simulink model "IID_nms_2Dmodel_for"  (R2016b)
settings: Solver=ode15s  StartTime=0.0  StopTime=t_end  FixedStep=1e-3  MaxStep=ts_max  RelTol=1e-3  AbsTol=1e-4  EnableMultiTasking=on
InitFcn:
  | IID_runScripts;
values from neighbouring files (symbols this model uses):
  D12_F = 0.16    [IID_nms_MechInit.m]    (also in nms_MechInit.m)
  D12_S = L_S    (= 0.5)    [IID_nms_MechInit.m]    (also in nms_MechInit.m = 0.46)
  D12_T = L_T    (= 0.5)    [IID_nms_MechInit.m]    (also in nms_MechInit.m = 0.46)
  D13_F = 0.20    (= 0.2)    [IID_nms_MechInit.m]    (also in nms_MechInit.m)
  D1G_F = 0.14    [IID_nms_MechInit.m]    (also in nms_MechInit.m)
  D1G_HAT = 0.35    [IID_nms_MechInit.m]    (also in nms_MechInit.m)
  D1G_S = 0.3    [IID_nms_MechInit.m]    (also in nms_MechInit.m = 0.28)
  D1G_T = 0.3    [IID_nms_MechInit.m]    (also in nms_MechInit.m = 0.28)
  DeltaThRef = 5e-3    (= 0.005)    [IID_nms_MechInit.m]    (also in nms_MechInit.m)
  Dist_On = 1    [IID_setDistPar.m]    (also in setDistPar.m)
  Dist_PDur = 0.15    [IID_setDistPar.m]    (also in setDistPar.m)
  Dist_StartTime = 15    [IID_setDistPar.m]    (also in setDistPar.m)
  Dist_xyzHAT_sag_PH = 0    [IID_setDistPar.m]    (also in setDistPar.m)
  In_F = 0.005    [IID_nms_MechInit.m]    (also in nms_MechInit.m)
  In_HAT = 3    [IID_nms_MechInit.m]    (also in nms_MechInit.m = 2.5)
  In_S = 0.05    [IID_nms_MechInit.m]    (also in nms_MechInit.m)
  In_T = 0.15    [IID_nms_MechInit.m]    (also in nms_MechInit.m)
  k_gx = (2*(m_F+m_S+m_T)+m_HAT)*g/0.1    (= 7848)    [IID_nms_MechInit.m]
  k_gy = (2*(m_F+m_S+m_T)+m_HAT)*g/0.01    (= 78480)    [IID_nms_MechInit.m]
  k_pressure = m_HAT * 9.81 / DeltaThRef    (= 104967)    [IID_nms_MechInit.m]    (also in nms_MechInit.m)
  m_F = 1.25    [IID_nms_MechInit.m]    (also in nms_MechInit.m)
  m_HAT = 53.5    [IID_nms_MechInit.m]    (also in nms_MechInit.m)
  m_S = 3.5    [IID_nms_MechInit.m]    (also in nms_MechInit.m)
  m_T = 8.5    [IID_nms_MechInit.m]    (also in nms_MechInit.m)
  m_Total = m_F*2+m_S*2+m_T*2+m_HAT    (= 80)    [IID_nms_MechInit.m]    (also in nms_MechInit.m)
  MidDelay = 0.010    (= 0.01)    [IID_setCtrlPar.m]    (also in nms_MechInit.m = 0.005)
  mu_slide = 0.8    [IID_nms_MechInit.m]    (also in nms_MechInit.m)
  mu_stick = 0.9    [IID_nms_MechInit.m]    (also in nms_MechInit.m)
  N = 1.5    [IID_nms_MechInit.m]    (also in cmaes_parfor.m = size(x,1); nms_MechInit.m)
  s = x(1:N-1,:).^2 + x(2:N,:).^2    [cmaes_parfor.m]
  ThPos = 4/5    (= 0.8)    [IID_nms_MechInit.m]    (also in nms_MechInit.m)
  v_gx_max = 0.03    [IID_nms_MechInit.m]
  v_gy_max = 0.03    [IID_nms_MechInit.m]
  v_max_pressure = 0.5    [IID_nms_MechInit.m]    (also in nms_MechInit.m)
  vLimit = 0.01    [IID_nms_MechInit.m]    (also in nms_MechInit.m)
undefined symbols (not defined in the file or in its folder): sgn
libraries: mblibv1 x71, cpg_lib x23, simulink x21, simulink_extras x6
(part 1 of 3)
settings Model: SimulationMode=accelerator  Creator=hgeyer  LastModifiedBy=brugtjh
settings SolverCC: ZeroCrossControl=DisableAll
settings DataIOCC: SaveFormat=Array  SignalLoggingSaveFormat=ModelDataLogs  SignalLogging=off
settings OptimizationCC: BooleanDataType=off  ExpressionDepthLimit=2147483647  InitFltsAndDblsToZero=on  EfficientMapNaN2IntZero=off  LifeSpan=inf
settings DebuggingCC: SaveWithParameterizedLinksMsg=none  UnderspecifiedInitializationDetection=Classic  MergeDetectMultiDrivingBlocksExec=none  SignalResolutionControl=TryResolveAllWithWarning  SolverPrmCheckMsg=warning  MultiTaskDSMMsg=warning  MultiTaskCondExecSysMsg=none  FcnCallInpInsideContextMsg=warning  AllowSymbolicDim=off  StateNameClashWarn=warning  SFUnexpectedBacktrackingDiag=warning  SFNoUnconditionalDefaultTransitionDiag=warning  SFExecutionAtInitializationDiag=none
settings HardwareCC: ProdBitPerPointer=32  ProdBitPerSizeT=32  ProdBitPerPtrDiffT=32  ProdLargestAtomicFloat=None  ProdIntDivRoundTo=Undefined  ProdEndianess=Unspecified  ProdWordSize=32  ProdHWDeviceType=32-bit Generic  TargetBitPerPointer=64  TargetBitPerSizeT=64  TargetBitPerPtrDiffT=64  TargetLongLongMode=on  TargetIntDivRoundTo=Zero  TargetEndianess=LittleEndian  TargetWordSize=64  TargetHWDeviceType=MATLAB Host  ProdEqTarget=off
settings ModelReferenceCC: PropagateSignalLabelsOutOfModel=off
settings CodeAppCC: MaxIdLength=128
settings GRTTargetCC: TargetLangStandard=C89/C90 (ANSI)  CombineOutputUpdateFcns=off  GRTInterface=on
settings ConfigComp: CovMetricSettings=dw  CovHtmlReporting=on  CovSaveCumulativeToWorkspaceVar=on  CovSaveSingleToWorkspaceVar=on  CovExternalEMLEnable=off
settings ConfigurationSet: Description=SimMechanics 2G
settings ExplorerConfigSet: SimMechanicsOpenEditorOnUpdate=off

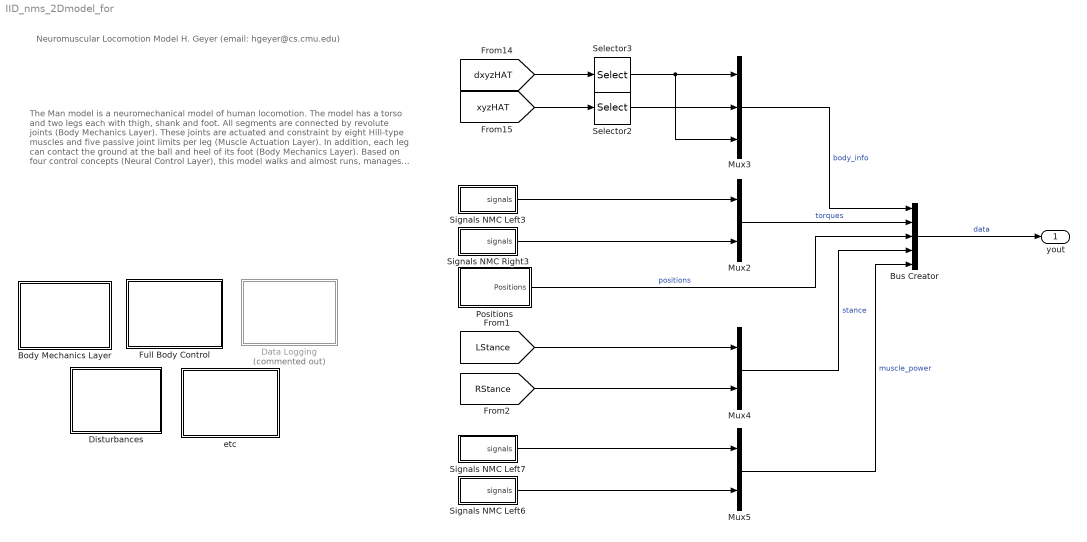
== system IID_nms_2Dmodel_for ==
  note: The Man model is a neuromechanical model of human locomotion.
      | The model has a torso and two legs each with thigh, shank and
      | foot. All segments are connected by revolute joints (Body Mechanics
      | Layer). These joints are actuated and constraint by eight Hill-type
      | muscles and five passive joint limits per leg (Muscle Actuation Layer).
      | In addition, each leg can contact the ground at the ball and heel of
      | its foot (Body Mechanics Layer).
      |
      | Based on four control concepts (Neural Control Layer), this
      | model walks and almost runs, manages slopes and random ground
      | levels, and adapts to different surfaces.
  note: Neuromuscular Locomotion Model
      | H. Geyer
      | (email: hgeyer@cs.cmu.edu)
  Body Mechanics Layer : Subsystem
  Bus Creator : BusCreator  Inputs=5
  Data Logging : Subsystem  Commented=on
  Disturbances : Subsystem
  Full Body Control : Subsystem
  Mux2 : Mux  Inputs=2
  Mux3 : Mux  Inputs=3
  Mux4 : Mux  Inputs=2
  Mux5 : Mux  Inputs=2
  Positions : Subsystem
  Selector2 : Selector  InputPortWidth=3  IndexOptions=Index vector (dialog)  Indices=[1]  OutputSizes=1
  Selector3 : Selector  InputPortWidth=3  IndexOptions=Index vector (dialog)  Indices=[1]  OutputSizes=1
  Signals NMC Left3 : Subsystem
  Signals NMC Left6 : Subsystem
  Signals NMC Left7 : Subsystem
  Signals NMC Right3 : Subsystem
  etc : Subsystem
  yout : Outport
  wires:
  Bus Creator/1 -> yout/1  "data"
  Selector3/1 -> Mux3/3, Mux3/1
  [dxyzHAT] -> Selector3/1
  [xyzHAT] -> Selector2/1
  Selector2/1 -> Mux3/2
  Mux3/1 -> Bus Creator/1  "body_info"
  Signals NMC Left3/1(signals) -> Mux2/1
  Signals NMC Right3/1(signals) -> Mux2/2
  Mux2/1 -> Bus Creator/2  "torques"
  Positions/1(Positions) -> Bus Creator/3  "positions"
  [LStance] -> Mux4/1
  [RStance] -> Mux4/2
  Mux4/1 -> Bus Creator/4  "stance"
  Signals NMC Left6/1(signals) -> Mux5/2
  Signals NMC Left7/1(signals) -> Mux5/1
  Mux5/1 -> Bus Creator/5  "muscle_power"

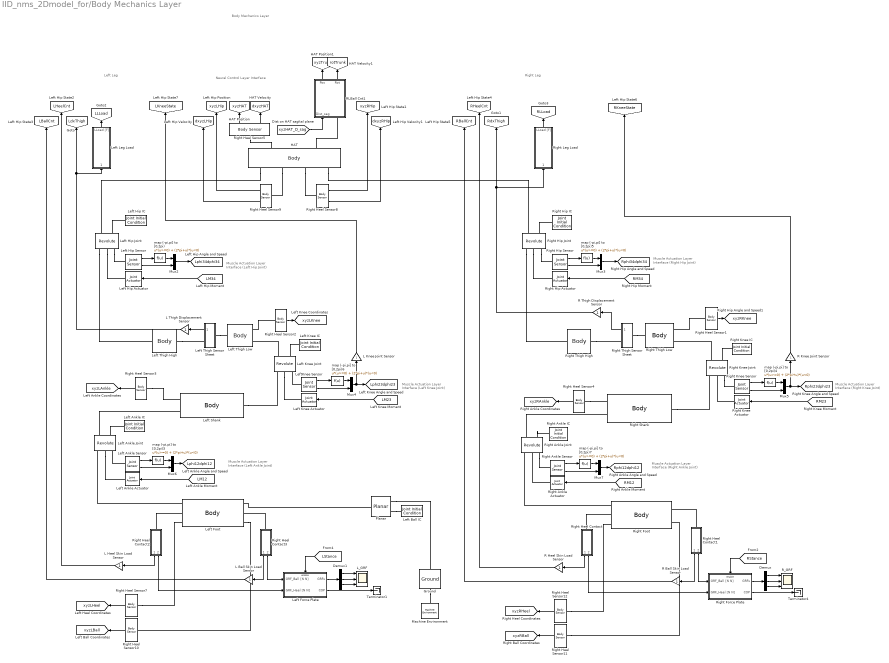
== system IID_nms_2Dmodel_for/Body Mechanics Layer ==
  note: Body Mechanics Layer
  note: Left Leg
  note: Right Leg
  note: Muscle Actuation
      | Layer Interface
      | (Left Hip Joint)
  note: Muscle Actuation
      | Layer Interface
      | (Right Hip Joint)
  note: Muscle Actuation
      | Layer Interface
      | (Right Knee Joint)
  note: Muscle Actuation
      | Layer Interface
      | (Left Knee Joint)
  note: Muscle Actuation
      | Layer Interface
      | (Left Ankle Joint)
  note: Muscle Actuation
      | Layer Interface
      | (Right Ankle Joint)
  note: Neural Control Layer Interface
  Demux : Demux  Outputs=3
  Demux1 : Demux  Outputs=3
  Ground : mblibv1/Bodies/Ground  UpdateFromCAD=off  LeftPortType=env  RightPortType=workingframe  PhysicalDomain=Mechanical  DialogClass=GroundBlock  CoordPosition=[0 0 0]  CoordPositionUnits=m  StateVectorMgrId=-1  MachineId=[0 0]  ShowEnvPort=on  ParameterChecksum=[3274320975, 1670571099, 3302951954, 713231611]  TopologyChecksum=[2253370739, 2650906436, 1237763067, 2817762160]
  HAT : mblibv1/Bodies/Body  LConnTagsString=CG|CS6  RConnTagsString=CS1|CS2|CS3|CS4  UpdateFromCAD=off  DialogClass=MechanicalBodyBlock  Mass=m_HAT  MassUnits=kg  InertiaUnits=kg*m^2  Inertia=In_HAT*[0 0 0; 0 0 0; 0 0 1]  Shape=Cylinder  ShapeDims=[1 1]  ShapeUnits=m  ShapeUse=false  Density=1  DensityUnits=kg/m^3  DensityUse=false  GraphicsMode=MACHINE_DEFAULT  BodyColorSelMode=MACHINE_DEFAULT  BodyColor=[1 0 0]  AttachedToCS=CG  CG=Left$CG$[D1G_HAT 0 0]$CS1$CS1$m$[0 0 0]$Euler X-Y-Z$deg$WORLD$true$none  WorkingFrames=Right$CS1$[0 0 0]$ADJOINING$ADJOINING$m$[0 0 0]$Euler X-Y-Z$deg$WORLD$true$none#Right$CS2$[0 0 0]$CS1$CS1$m$[0 0 0]$Euler X-Y-Z$deg$WORLD$true$none#Right$CS3$[0 0 0]$CS1$CS1$m$[0 0 0]$Euler X-Y-Z$deg$WORLD$true$none#Right$CS4$[0 0 0]$CS1$CS1$m$[0 0 0]$Euler X-Y-Z$deg$WORLD$true$none#Left$CS6$[0 0 0]$CS1$CS1$m$[0 0 0]$Euler X-Y-Z$deg$WORLD$true$none#Left$CS5$[2*D1G_HAT 0 0]$CS1$CS1$m$[0 0 0]$Euler X-Y-Z$deg$WORLD$false$none  CGPos=[D1G_HAT 0 0]  CGRot=[0 0 0]  CS0Pos=[]  CS0Rot=[]  CS1Pos=[0 0 0]  CS1Rot=[0 0 0]  CS2Pos=[0 0 0]  CS2Rot=[0 0 0]  CS3Pos=[0 0 0]  CS3Rot=[0 0 0]  CS4Pos=[0 0 0]  CS4Rot=[0 0 0]  CS5Pos=[2*D1G_HAT 0 0]  CS5Rot=[0 0 0]  CS6Pos=[0 0 0]  CS6Rot=[0 0 0]  CS7Pos=[]  CS7Rot=[]  CS8Pos=[]  CS8Rot=[]  CS9Pos=[]  CS9Rot=[]  CS10Pos=[]  CS10Rot=[]  CS11Pos=[]  CS11Rot=[]  CS12Pos=[]  CS12Rot=[]  CS13Pos=[]  CS13Rot=[]  CS14Pos=[]  CS14Rot=[]  CS15Pos=[]  CS15Rot=[]  CS16Pos=[]  CS16Rot=[]  CS17Pos=[]  CS17Rot=[]  CS18Pos=[]  CS18Rot=[]  CS19Pos=[]  CS19Rot=[]  CS20Pos=[]  CS20Rot=[]
  L Ball Skin Load Sensor : Gain
  L Heel Skin Load Sensor : Gain
  L Knee Joint Sensor : Gain
  L Thigh Displacement  Sensor : Gain
  L_GRF : Scope  NumInputPorts=3
  Left Ankle Joint : mblibv1/Joints/Revolute  LConnTagsString=__newl0|SA1|SA2  RConnTagsString=__newr0|SA1  UpdateFromCAD=off  NumSAPorts=3  CutJoint=off  MarkAsCut=off  Primitives=revolute  PrimitiveProps=R1$WORLD$[0 0 1]$revolute  DialogClass=JointBlock  R1Axis=[0 0 1]
  Left Hip Joint : mblibv1/Joints/Revolute  LConnTagsString=__newl0|SA1|SA2  RConnTagsString=__newr0|SA1  UpdateFromCAD=off  NumSAPorts=3  CutJoint=off  MarkAsCut=off  Primitives=revolute  PrimitiveProps=R1$WORLD$[0 0 1]$revolute  DialogClass=JointBlock  R1Axis=[0 0 1]
  Left Knee Joint : mblibv1/Joints/Revolute  LConnTagsString=__newl0|SA1|SA2  RConnTagsString=__newr0|SA1  UpdateFromCAD=off  NumSAPorts=3  CutJoint=off  MarkAsCut=off  Primitives=revolute  PrimitiveProps=R1$WORLD$[0 0 -1]$revolute  DialogClass=JointBlock  R1Axis=[0 0 -1]
  Left Ankle Actuator : mblibv1/Sensors &  Actuators/Joint Actuator  UpdateFromCAD=off  PhysicalDomain=Mechanical  PortType=blob  ActuationStyle=Force  AngleUnits=deg  ArcVelocityUnits=deg/s  ArcAccelerationUnits=deg/s^2  CoordPositionUnits=m  VelocityUnits=m/s  AccelerationUnits=m/s^2  ForceUnits=N  TorqueUnits=N-m  ActiveIO=on  Width=1  DialogClass=MechanicalActuatorBlock  Primitive=R1  ReferenceFrame=Absolute (INERTIAL)
  Left Ankle Sensor : mblibv1/Sensors &  Actuators/Joint Sensor  UpdateFromCAD=off  PhysicalDomain=Mechanical  PortType=blob  Muxed=off  Pose=off  Angle=on  AngleUnits=rad  ArcVelocity=on  ArcVelocityUnits=rad/s  ArcAcceleration=off  ArcAccelerationUnits=deg/s^2  CoordPosition=on  CoordPositionUnits=m  Velocity=off  VelocityUnits=m/s  Acceleration=off  AccelerationUnits=m/s^2  Quaternion=on  QuaternionDT=off  QuaternionDDT=off  QuaternionUnits=off  OutputVector=[ 1 1 ]  ActiveIO=on  Width=2  DialogClass=MechanicalSensorBlock  Primitive=R1  Force=off  ForceUnits=N  Torque=off  TorqueUnits=N-m  ReferenceFrame=Absolute (INERTIAL)  ReactionSensedSide=Base  ReactionReferenceFrame=Absolute (World)  ReactionForce=off  ReactionForceUnits=N  ReactionMoment=off  ReactionMomentUnits=N-m
  Left Ankle IC : mblibv1/Sensors &  Actuators/Joint Initial Condition  UpdateFromCAD=off  LeftPortType=blob  RightPortType=blob  PhysicalDomain=mechanical  DialogClass=InitialConditionBlock  InitialConditions=P1$false$0$m$rad$0$m/s$rad/s#P2$false$0$m$rad$0$m/s$rad/s#P3$false$0$m$rad$0$m/s$rad/s#R1$true$Lphi120$m$rad$0$m/s$rad/s#R2$false$0$m$rad$0$m/s$rad/s#R3$false$0$m$rad$0$m/s$rad/s#S$false$0$m$rad$0$m/s$rad/s  P1PIC=0  P1VIC=0  P2PIC=0  P2VIC=0  P3PIC=0  P3VIC=0  R1PIC=Lphi120  R1VIC=0  R2PIC=0  R2VIC=0  R3PIC=0  R3VIC=0  SPIC=0  SVIC=0
  Left Ball IC : mblibv1/Sensors &  Actuators/Joint Initial Condition  UpdateFromCAD=off  LeftPortType=blob  RightPortType=blob  PhysicalDomain=Mechanical  DialogClass=InitialConditionBlock  InitialConditions=P1$true$0$m$rad$vx0$m/s$rad/s#P2$true$0$m$rad$0$m/s$rad/s#P3$false$0$m$rad$0$m/s$rad/s#R1$false$0$m$rad$0$m/s$rad/s#R2$false$0$m$rad$0$m/s$rad/s#R3$false$0$m$rad$0$m/s$rad/s#S$false$0$m$rad$0$m/s$rad/s  P1PIC=0  P1VIC=vx0  P2PIC=0  P2VIC=0  P3PIC=0  P3VIC=0  R1PIC=0  R1VIC=0  R2PIC=0  R2VIC=0  R3PIC=0  R3VIC=0  SPIC=0  SVIC=0
  Left Foot : mblibv1/Bodies/Body  LConnTagsString=CS1|CS4|CS6  RConnTagsString=CS2|CS3|CS5  UpdateFromCAD=off  DialogClass=MechanicalBodyBlock  Mass=m_F  MassUnits=kg  InertiaUnits=kg*m^2  Inertia=[0 0 0; 0 0 0; 0 0 In_F]  Shape=Cylinder  ShapeDims=[1 1]  ShapeUnits=m  ShapeUse=false  Density=1  DensityUnits=kg/m^3  DensityUse=false  GraphicsMode=MACHINE_DEFAULT  BodyColorSelMode=MACHINE_DEFAULT  BodyColor=[1 0 0]  AttachedToCS=CG  CG=Left$CG$[-D1G_F 0 0]$CS1$CS1$m$[0 0 0]$Euler X-Y-Z$deg$WORLD$false$none  WorkingFrames=Left$CS1$[0 0 0]$ADJOINING$ADJOINING$m$[0 0 0]$Euler X-Y-Z$deg$WORLD$true$none#Right$CS2$[-D12_F 0 0]$CS1$CS1$m$[0 0 0]$Euler X-Y-Z$deg$WORLD$true$none#Right$CS3$[-D13_F 0 0]$CS1$CS1$m$[0 0 0]$Euler X-Y-Z$deg$WORLD$true$none#Right$CS5$[0 0 0]$CS3$CS3$m$[0 0 0]$Euler X-Y-Z$deg$WORLD$true$none#Left$CS4$[0 0 0]$CS1$CS1$m$[0 0 0]$Euler X-Y-Z$deg$WORLD$true$none#Left$CS6$[0 0 0]$CS4$CS4$m$[0 0 0]$Euler X-Y-Z$deg$WORLD$true$none  CGPos=[-D1G_F 0 0]  CGRot=[0 0 0]  CS0Pos=[]  CS0Rot=[]  CS1Pos=[0 0 0]  CS1Rot=[0 0 0]  CS2Pos=[-D12_F 0 0]  CS2Rot=[0 0 0]  CS3Pos=[-D13_F 0 0]  CS3Rot=[0 0 0]  CS4Pos=[0 0 0]  CS4Rot=[0 0 0]  CS5Pos=[0 0 0]  CS5Rot=[0 0 0]  CS6Pos=[0 0 0]  CS6Rot=[0 0 0]  CS7Pos=[]  CS7Rot=[]  CS8Pos=[]  CS8Rot=[]  CS9Pos=[]  CS9Rot=[]  CS10Pos=[]  CS10Rot=[]  CS11Pos=[]  CS11Rot=[]  CS12Pos=[]  CS12Rot=[]  CS13Pos=[]  CS13Rot=[]  CS14Pos=[]  CS14Rot=[]  CS15Pos=[]  CS15Rot=[]  CS16Pos=[]  CS16Rot=[]  CS17Pos=[]  CS17Rot=[]  CS18Pos=[]  CS18Rot=[]  CS19Pos=[]  CS19Rot=[]  CS20Pos=[]  CS20Rot=[]
  Left Force Plate : Subsystem  TreatAsAtomicUnit=on
  Left Hip Actuator : mblibv1/Sensors &  Actuators/Joint Actuator  UpdateFromCAD=off  PhysicalDomain=Mechanical  PortType=blob  ActuationStyle=Force  AngleUnits=deg  ArcVelocityUnits=deg/s  ArcAccelerationUnits=deg/s^2  CoordPositionUnits=m  VelocityUnits=m/s  AccelerationUnits=m/s^2  ForceUnits=N  TorqueUnits=N-m  ActiveIO=on  Width=1  DialogClass=MechanicalActuatorBlock  Primitive=R1  ReferenceFrame=Absolute (INERTIAL)
  Left Hip Sensor : mblibv1/Sensors &  Actuators/Joint Sensor  UpdateFromCAD=off  PhysicalDomain=Mechanical  PortType=blob  Muxed=off  Pose=off  Angle=on  AngleUnits=rad  ArcVelocity=on  ArcVelocityUnits=rad/s  ArcAcceleration=off  ArcAccelerationUnits=deg/s^2  CoordPosition=on  CoordPositionUnits=m  Velocity=on  VelocityUnits=m/s  Acceleration=off  AccelerationUnits=m/s^2  Quaternion=on  QuaternionDT=off  QuaternionDDT=off  QuaternionUnits=off  OutputVector=[ 1 1 ]  ActiveIO=on  Width=2  DialogClass=MechanicalSensorBlock  Primitive=R1  Force=off  ForceUnits=N  Torque=off  TorqueUnits=N-m  ReferenceFrame=Absolute (INERTIAL)  ReactionSensedSide=Base  ReactionReferenceFrame=Absolute (World)  ReactionForce=off  ReactionForceUnits=N  ReactionMoment=off  ReactionMomentUnits=N-m
  Left Hip IC : mblibv1/Sensors &  Actuators/Joint Initial Condition  UpdateFromCAD=off  LeftPortType=blob  RightPortType=blob  PhysicalDomain=mechanical  DialogClass=InitialConditionBlock  InitialConditions=P1$false$0$m$rad$0$m/s$rad/s#P2$false$0$m$rad$0$m/s$rad/s#P3$false$0$m$rad$0$m/s$rad/s#R1$true$Lphi340$m$rad$0$m/s$rad/s#R2$false$0$m$rad$0$m/s$rad/s#R3$false$0$m$rad$0$m/s$rad/s#S$false$0$m$rad$0$m/s$rad/s  P1PIC=0  P1VIC=0  P2PIC=0  P2VIC=0  P3PIC=0  P3VIC=0  R1PIC=Lphi340  R1VIC=0  R2PIC=0  R2VIC=0  R3PIC=0  R3VIC=0  SPIC=0  SVIC=0
  Left Knee Actuator : mblibv1/Sensors &  Actuators/Joint Actuator  UpdateFromCAD=off  PhysicalDomain=Mechanical  PortType=blob  ActuationStyle=Force  AngleUnits=deg  ArcVelocityUnits=deg/s  ArcAccelerationUnits=deg/s^2  CoordPositionUnits=m  VelocityUnits=m/s  AccelerationUnits=m/s^2  ForceUnits=N  TorqueUnits=N-m  ActiveIO=on  Width=1  DialogClass=MechanicalActuatorBlock  Primitive=R1  ReferenceFrame=Absolute (INERTIAL)
  Left Knee IC : mblibv1/Sensors &  Actuators/Joint Initial Condition  UpdateFromCAD=off  LeftPortType=blob  RightPortType=blob  PhysicalDomain=mechanical  DialogClass=InitialConditionBlock  InitialConditions=P1$false$0$m$rad$0$m/s$rad/s#P2$false$0$m$rad$0$m/s$rad/s#P3$false$0$m$rad$0$m/s$rad/s#R1$true$Lphi230$m$rad$0$m/s$deg/s#R2$false$0$m$rad$0$m/s$rad/s#R3$false$0$m$rad$0$m/s$rad/s#S$false$0$m$rad$0$m/s$rad/s  P1PIC=0  P1VIC=0  P2PIC=0  P2VIC=0  P3PIC=0  P3VIC=0  R1PIC=Lphi230  R1VIC=0  R2PIC=0  R2VIC=0  R3PIC=0  R3VIC=0  SPIC=0  SVIC=0
  Left Leg Load : Subsystem
  Left Shank : mblibv1/Bodies/Body  LConnTagsString=CS3|CS1  RConnTagsString=CS2  UpdateFromCAD=off  DialogClass=MechanicalBodyBlock  Mass=m_S  MassUnits=kg  InertiaUnits=kg*m^2  Inertia=[0 0 0; 0 0 0; 0 0 In_S]  Shape=Cylinder  ShapeDims=[1 1]  ShapeUnits=m  ShapeUse=false  Density=1  DensityUnits=kg/m^3  DensityUse=false  GraphicsMode=MACHINE_DEFAULT  BodyColorSelMode=MACHINE_DEFAULT  BodyColor=[1 0 0]  AttachedToCS=CG  CG=Left$CG$[D1G_S 0 0]$CS1$CS1$m$[0 0 0]$Euler X-Y-Z$deg$WORLD$false$none  WorkingFrames=Left$CS3$[0 0 0]$CS1$CS1$m$[0 0 0]$Euler X-Y-Z$deg$WORLD$true$none#Left$CS1$[0 0 0]$ADJOINING$ADJOINING$m$[0 0 0]$Euler X-Y-Z$deg$WORLD$true$none#Right$CS2$[D12_S 0 0]$CS1$CS1$m$[0 0 0]$Euler X-Y-Z$deg$WORLD$true$none  CGPos=[D1G_S 0 0]  CGRot=[0 0 0]  CS0Pos=[]  CS0Rot=[]  CS1Pos=[0 0 0]  CS1Rot=[0 0 0]  CS2Pos=[D12_S 0 0]  CS2Rot=[0 0 0]  CS3Pos=[0 0 0]  CS3Rot=[0 0 0]  CS4Pos=[]  CS4Rot=[]  CS5Pos=[]  CS5Rot=[]  CS6Pos=[]  CS6Rot=[]  CS7Pos=[]  CS7Rot=[]  CS8Pos=[]  CS8Rot=[]  CS9Pos=[]  CS9Rot=[]  CS10Pos=[]  CS10Rot=[]  CS11Pos=[]  CS11Rot=[]  CS12Pos=[]  CS12Rot=[]  CS13Pos=[]  CS13Rot=[]  CS14Pos=[]  CS14Rot=[]  CS15Pos=[]  CS15Rot=[]  CS16Pos=[]  CS16Rot=[]  CS17Pos=[]  CS17Rot=[]  CS18Pos=[]  CS18Rot=[]  CS19Pos=[]  CS19Rot=[]  CS20Pos=[]  CS20Rot=[]
  Left Thigh Sensor Sheet : Subsystem
  Left Thigh High : mblibv1/Bodies/Body  LConnTagsString=CS2  RConnTagsString=CS1  UpdateFromCAD=off  DialogClass=MechanicalBodyBlock  Mass=m_T*(1-ThPos)  MassUnits=kg  InertiaUnits=kg*m^2  Inertia=[0 0 0; 0 0 0; 0 0 In_T*(1-ThPos)^3]  Shape=Cylinder  ShapeDims=[1 1]  ShapeUnits=m  ShapeUse=false  Density=1  DensityUnits=kg/m^3  DensityUse=false  GraphicsMode=MACHINE_DEFAULT  BodyColorSelMode=MACHINE_DEFAULT  BodyColor=[1;0;0]  AttachedToCS=CG  CG=Left$CG$[-D1G_T*(1-ThPos) 0 0]$CS1$CS1$m$[0 0 0]$Euler X-Y-Z$deg$WORLD$false  WorkingFrames=Right$CS1$[0 0 0]$ADJOINING$ADJOINING$m$[0 0 0]$Euler X-Y-Z$deg$WORLD$true#Left$CS2$[-D12_T*(1-ThPos) 0 0]$CS1$CS1$m$[0 0 0]$Euler X-Y-Z$deg$WORLD$true  CGPos=[-D1G_T*(1-ThPos) 0 0]  CGRot=[0 0 0]  CS0Pos=[]  CS0Rot=[]  CS1Pos=[0 0 0]  CS1Rot=[0 0 0]  CS2Pos=[-D12_T*(1-ThPos) 0 0]  CS2Rot=[0 0 0]  CS3Pos=[]  CS3Rot=[]  CS4Pos=[]  CS4Rot=[]  CS5Pos=[]  CS5Rot=[]  CS6Pos=[]  CS6Rot=[]  CS7Pos=[]  CS7Rot=[]  CS8Pos=[]  CS8Rot=[]  CS9Pos=[]  CS9Rot=[]  CS10Pos=[]  CS10Rot=[]  CS11Pos=[]  CS11Rot=[]  CS12Pos=[]  CS12Rot=[]  CS13Pos=[]  CS13Rot=[]  CS14Pos=[]  CS14Rot=[]  CS15Pos=[]  CS15Rot=[]  CS16Pos=[]  CS16Rot=[]  CS17Pos=[]  CS17Rot=[]  CS18Pos=[]  CS18Rot=[]  CS19Pos=[]  CS19Rot=[]  CS20Pos=[]  CS20Rot=[]
  Left Thigh Low : mblibv1/Bodies/Body  LConnTagsString=CS2  RConnTagsString=CS3|CS1  UpdateFromCAD=off  DialogClass=MechanicalBodyBlock  Mass=m_T*ThPos  MassUnits=kg  InertiaUnits=kg*m^2  Inertia=[0 0 0; 0 0 0; 0 0 In_T*(ThPos)^3]  Shape=Cylinder  ShapeDims=[1 1]  ShapeUnits=m  ShapeUse=false  Density=1  DensityUnits=kg/m^3  DensityUse=false  GraphicsMode=MACHINE_DEFAULT  BodyColorSelMode=MACHINE_DEFAULT  BodyColor=[1 0 0]  AttachedToCS=CG  CG=Left$CG$[-D1G_T*ThPos 0 0]$CS1$CS1$m$[0 0 0]$Euler X-Y-Z$deg$WORLD$false$none  WorkingFrames=Right$CS3$[0 0 0]$CS1$CS1$m$[0 0 0]$Euler X-Y-Z$deg$WORLD$true$none#Right$CS1$[0 0 0]$ADJOINING$ADJOINING$m$[0 0 0]$Euler X-Y-Z$deg$WORLD$true$none#Left$CS2$[-D12_T*ThPos 0 0]$CS1$CS1$m$[0 0 0]$Euler X-Y-Z$deg$WORLD$true$none  CGPos=[-D1G_T*ThPos 0 0]  CGRot=[0 0 0]  CS0Pos=[]  CS0Rot=[]  CS1Pos=[0 0 0]  CS1Rot=[0 0 0]  CS2Pos=[-D12_T*ThPos 0 0]  CS2Rot=[0 0 0]  CS3Pos=[0 0 0]  CS3Rot=[0 0 0]  CS4Pos=[]  CS4Rot=[]  CS5Pos=[]  CS5Rot=[]  CS6Pos=[]  CS6Rot=[]  CS7Pos=[]  CS7Rot=[]  CS8Pos=[]  CS8Rot=[]  CS9Pos=[]  CS9Rot=[]  CS10Pos=[]  CS10Rot=[]  CS11Pos=[]  CS11Rot=[]  CS12Pos=[]  CS12Rot=[]  CS13Pos=[]  CS13Rot=[]  CS14Pos=[]  CS14Rot=[]  CS15Pos=[]  CS15Rot=[]  CS16Pos=[]  CS16Rot=[]  CS17Pos=[]  CS17Rot=[]  CS18Pos=[]  CS18Rot=[]  CS19Pos=[]  CS19Rot=[]  CS20Pos=[]  CS20Rot=[]
  LeftKnee Sensor : mblibv1/Sensors &  Actuators/Joint Sensor  UpdateFromCAD=off  PhysicalDomain=Mechanical  PortType=blob  Muxed=off  Pose=off  Angle=on  AngleUnits=rad  ArcVelocity=on  ArcVelocityUnits=rad/s  ArcAcceleration=off  ArcAccelerationUnits=deg/s^2  CoordPosition=on  CoordPositionUnits=m  Velocity=off  VelocityUnits=m/s  Acceleration=off  AccelerationUnits=m/s^2  Quaternion=on  QuaternionDT=off  QuaternionDDT=off  QuaternionUnits=off  OutputVector=[ 1 1 ]  ActiveIO=on  Width=2  DialogClass=MechanicalSensorBlock  Primitive=R1  Force=off  ForceUnits=N  Torque=off  TorqueUnits=N-m  ReferenceFrame=Absolute (INERTIAL)  ReactionSensedSide=Base  ReactionReferenceFrame=Absolute (World)  ReactionForce=off  ReactionForceUnits=N  ReactionMoment=off  ReactionMomentUnits=N-m
  Machine Environment : mblibv1/Bodies/Machine Environment  Tag=Factory ground  PortType=env  PhysicalDomain=Mechanical  DialogTemplateClass=MECH.MachineEnvironment  SyncWhenCopied=off  Gravity=[0 -9.81 0]  GravityUnits=m/s^2  GravityAsSignal=off  Dimensionality=2D Only  AnalysisType=Forward dynamics  LinearAssemblyTolerance=1e-3  LinearAssemblyToleranceUnits=m  AngularAssemblyTolerance=1e-3  AngularAssemblyToleranceUnits=rad  ConstraintSolverType=Tolerancing  ConstraintRelTolerance=1e-3  ConstraintAbsTolerance=1e-3  UseRobustSingularityHandling=off  RedundancyAnalysisToleranceType=Automatically select tolerance  RedundancyAnalysisTolerance=1e-14  StatePerturbationType=Fixed  PerturbationSize=1e-3  VisualizeMachine=on  BodyVisualizationType=Use model default body geometries  BodyColorSelMode=Use model default  DefaultBodyColor=[1 0 0]
  Mux{2..7} (6 alike) : Mux  Inputs=2
  Planar : mblibv1/Joints/Planar  LConnTagsString=__newl0|SA1  RConnTagsString=__newr0  UpdateFromCAD=off  NumSAPorts=1  CutJoint=off  MarkAsCut=off  Primitives=prismatic_prismatic_revolute  PrimitiveProps=P1$WORLD$[1 0 0]$prismatic#P2$WORLD$[0 1 0]$prismatic#R1$WORLD$[0 0 1]$revolute  DialogClass=JointBlock  P1Axis=[1 0 0]  P2Axis=[0 1 0]  R1Axis=[0 0 1]
  R Ball Skin Load Sensor : Gain
  R Heel Skin Load Sensor : Gain
  R Knee Joint Sensor : Gain
  R Thigh Displacement  Sensor : Gain
  RLBall Cnt1 : Subsystem
  R_GRF : Scope  NumInputPorts=3
  Right Ankle Joint : mblibv1/Joints/Revolute  LConnTagsString=__newl0|SA1|SA2  RConnTagsString=__newr0|SA1  UpdateFromCAD=off  NumSAPorts=3  CutJoint=off  MarkAsCut=off  Primitives=revolute  PrimitiveProps=R1$WORLD$[0 0 1]$revolute  DialogClass=JointBlock  R1Axis=[0 0 1]
  Right Heel Contact : Subsystem
  Right Heel Contact1 : Subsystem
  Right Heel Contact2 : Subsystem
  Right Heel Contact3 : Subsystem
  Right Hip Joint : mblibv1/Joints/Revolute  LConnTagsString=__newl0|SA1|SA2  RConnTagsString=__newr0|SA1  UpdateFromCAD=off  NumSAPorts=3  CutJoint=off  MarkAsCut=off  Primitives=revolute  PrimitiveProps=R1$WORLD$[0 0 1]$revolute  DialogClass=JointBlock  R1Axis=[0 0 1]
  Right Knee Joint : mblibv1/Joints/Revolute  LConnTagsString=__newl0|SA1|SA2  RConnTagsString=__newr0|SA1  UpdateFromCAD=off  NumSAPorts=3  CutJoint=off  MarkAsCut=off  Primitives=revolute  PrimitiveProps=R1$WORLD$[0 0 -1]$revolute  DialogClass=JointBlock  R1Axis=[0 0 -1]
  Right Ankle Actuator : mblibv1/Sensors &  Actuators/Joint Actuator  UpdateFromCAD=off  PhysicalDomain=Mechanical  PortType=blob  ActuationStyle=Force  AngleUnits=deg  ArcVelocityUnits=deg/s  ArcAccelerationUnits=deg/s^2  CoordPositionUnits=m  VelocityUnits=m/s  AccelerationUnits=m/s^2  ForceUnits=N  TorqueUnits=N-m  ActiveIO=on  Width=1  DialogClass=MechanicalActuatorBlock  Primitive=R1  ReferenceFrame=Absolute (INERTIAL)
  Right Ankle Sensor : mblibv1/Sensors &  Actuators/Joint Sensor  UpdateFromCAD=off  PhysicalDomain=Mechanical  PortType=blob  Muxed=off  Pose=off  Angle=on  AngleUnits=rad  ArcVelocity=on  ArcVelocityUnits=rad/s  ArcAcceleration=off  ArcAccelerationUnits=deg/s^2  CoordPosition=on  CoordPositionUnits=m  Velocity=off  VelocityUnits=m/s  Acceleration=off  AccelerationUnits=m/s^2  Quaternion=on  QuaternionDT=off  QuaternionDDT=off  QuaternionUnits=off  OutputVector=[ 1 1 ]  ActiveIO=on  Width=2  DialogClass=MechanicalSensorBlock  Primitive=R1  Force=off  ForceUnits=N  Torque=off  TorqueUnits=N-m  ReferenceFrame=Absolute (INERTIAL)  ReactionSensedSide=Base  ReactionReferenceFrame=Absolute (World)  ReactionForce=off  ReactionForceUnits=N  ReactionMoment=off  ReactionMomentUnits=N-m
  Right Ankle IC : mblibv1/Sensors &  Actuators/Joint Initial Condition  UpdateFromCAD=off  LeftPortType=blob  RightPortType=blob  PhysicalDomain=mechanical  DialogClass=InitialConditionBlock  InitialConditions=P1$false$0$m$rad$0$m/s$rad/s#P2$false$0$m$rad$0$m/s$rad/s#P3$false$0$m$rad$0$m/s$rad/s#R1$true$Rphi120$m$rad$0$m/s$rad/s#R2$false$0$m$rad$0$m/s$rad/s#R3$false$0$m$rad$0$m/s$rad/s#S$false$0$m$rad$0$m/s$rad/s  P1PIC=0  P1VIC=0  P2PIC=0  P2VIC=0  P3PIC=0  P3VIC=0  R1PIC=Rphi120  R1VIC=0  R2PIC=0  R2VIC=0  R3PIC=0  R3VIC=0  SPIC=0  SVIC=0
  Right Foot : mblibv1/Bodies/Body  LConnTagsString=CS1|CS5  RConnTagsString=CS2|CS3|CS4  UpdateFromCAD=off  DialogClass=MechanicalBodyBlock  Mass=m_F  MassUnits=kg  InertiaUnits=kg*m^2  Inertia=[0 0 0; 0 0 0; 0 0 In_F]  Shape=Cylinder  ShapeDims=[1 1]  ShapeUnits=m  ShapeUse=false  Density=1  DensityUnits=kg/m^3  DensityUse=false  GraphicsMode=MACHINE_DEFAULT  BodyColorSelMode=MACHINE_DEFAULT  BodyColor=[1 0 0]  AttachedToCS=CG  CG=Left$CG$[-D1G_F 0 0]$CS1$CS1$m$[0 0 0]$Euler X-Y-Z$deg$WORLD$false$none  WorkingFrames=Left$CS1$[0 0 0]$ADJOINING$ADJOINING$m$[0 0 0]$Euler X-Y-Z$deg$WORLD$true$none#Left$CS5$[0 0 0]$CS1$CS1$m$[0 0 0]$Euler X-Y-Z$deg$WORLD$true$none#Right$CS2$[-D12_F 0 0]$CS1$CS1$m$[0 0 0]$Euler X-Y-Z$deg$WORLD$true$none#Right$CS3$[-D13_F 0 0]$CS1$CS1$m$[0 0 0]$Euler X-Y-Z$deg$WORLD$true$none#Right$CS4$[0 0 0]$CS3$CS3$m$[0 0 0]$Euler X-Y-Z$deg$WORLD$true$none  CGPos=[-D1G_F 0 0]  CGRot=[0 0 0]  CS0Pos=[]  CS0Rot=[]  CS1Pos=[0 0 0]  CS1Rot=[0 0 0]  CS2Pos=[-D12_F 0 0]  CS2Rot=[0 0 0]  CS3Pos=[-D13_F 0 0]  CS3Rot=[0 0 0]  CS4Pos=[0 0 0]  CS4Rot=[0 0 0]  CS5Pos=[0 0 0]  CS5Rot=[0 0 0]  CS6Pos=[]  CS6Rot=[]  CS7Pos=[]  CS7Rot=[]  CS8Pos=[]  CS8Rot=[]  CS9Pos=[]  CS9Rot=[]  CS10Pos=[]  CS10Rot=[]  CS11Pos=[]  CS11Rot=[]  CS12Pos=[]  CS12Rot=[]  CS13Pos=[]  CS13Rot=[]  CS14Pos=[]  CS14Rot=[]  CS15Pos=[]  CS15Rot=[]  CS16Pos=[]  CS16Rot=[]  CS17Pos=[]  CS17Rot=[]  CS18Pos=[]  CS18Rot=[]  CS19Pos=[]  CS19Rot=[]  CS20Pos=[]  CS20Rot=[]
  Right Force Plate : Subsystem  TreatAsAtomicUnit=on
  Right Heel Sensor{1..4,7,10..12} (8 alike) : mblibv1/Sensors &  Actuators/Body Sensor  UpdateFromCAD=off  PhysicalDomain=Mechanical  PortType=blob  Muxed=off  Pose=off  Angle=on  AngleUnits=deg  ArcVelocity=off  ArcVelocityUnits=deg/s  ArcAcceleration=off  ArcAccelerationUnits=deg/s^2  CoordPosition=on  CoordPositionUnits=m  Velocity=off  VelocityUnits=m/s  Acceleration=off  AccelerationUnits=m/s^2  Quaternion=on  QuaternionDT=off  QuaternionDDT=off  QuaternionUnits=off  OutputVector=[ 3 3 ]  ActiveIO=on  Width=3  DialogClass=MechanicalSensorBlock  ReferenceFrame=Absolute (World)
  Right Heel Sensor5 : mblibv1/Sensors &  Actuators/Body Sensor  UpdateFromCAD=off  PhysicalDomain=Mechanical  PortType=blob  Muxed=off  Pose=off  Angle=on  AngleUnits=deg  ArcVelocity=off  ArcVelocityUnits=deg/s  ArcAcceleration=off  ArcAccelerationUnits=deg/s^2  CoordPosition=on  CoordPositionUnits=m  Velocity=on  VelocityUnits=m/s  Acceleration=off  AccelerationUnits=m/s^2  Quaternion=on  QuaternionDT=off  QuaternionDDT=off  QuaternionUnits=off  OutputVector=[ 3 3 ]  ActiveIO=on  Width=6  DialogClass=MechanicalSensorBlock  ReferenceFrame=Absolute (World)
  Right Heel Sensor8 : mblibv1/Sensors &  Actuators/Body Sensor  UpdateFromCAD=off  PhysicalDomain=Mechanical  PortType=blob  Muxed=off  Pose=off  Angle=on  AngleUnits=deg  ArcVelocity=off  ArcVelocityUnits=deg/s  ArcAcceleration=off  ArcAccelerationUnits=deg/s^2  CoordPosition=on  CoordPositionUnits=m  Velocity=on  VelocityUnits=m/s  Acceleration=off  AccelerationUnits=m/s^2  Quaternion=on  QuaternionDT=off  QuaternionDDT=off  QuaternionUnits=off  OutputVector=[ 3 3 ]  ActiveIO=on  Width=6  DialogClass=MechanicalSensorBlock  ReferenceFrame=Absolute (World)
  Right Heel Sensor9 : mblibv1/Sensors &  Actuators/Body Sensor  UpdateFromCAD=off  PhysicalDomain=Mechanical  PortType=blob  Muxed=off  Pose=off  Angle=on  AngleUnits=deg  ArcVelocity=off  ArcVelocityUnits=deg/s  ArcAcceleration=off  ArcAccelerationUnits=deg/s^2  CoordPosition=on  CoordPositionUnits=m  Velocity=on  VelocityUnits=m/s  Acceleration=off  AccelerationUnits=m/s^2  Quaternion=on  QuaternionDT=off  QuaternionDDT=off  QuaternionUnits=off  OutputVector=[ 3 3 ]  ActiveIO=on  Width=6  DialogClass=MechanicalSensorBlock  ReferenceFrame=Absolute (World)
  Right Hip Actuator : mblibv1/Sensors &  Actuators/Joint Actuator  UpdateFromCAD=off  PhysicalDomain=Mechanical  PortType=blob  ActuationStyle=Force  AngleUnits=deg  ArcVelocityUnits=deg/s  ArcAccelerationUnits=deg/s^2  CoordPositionUnits=m  VelocityUnits=m/s  AccelerationUnits=m/s^2  ForceUnits=N  TorqueUnits=N-m  ActiveIO=on  Width=1  DialogClass=MechanicalActuatorBlock  Primitive=R1  ReferenceFrame=Absolute (INERTIAL)
  Right Hip Sensor : mblibv1/Sensors &  Actuators/Joint Sensor  UpdateFromCAD=off  PhysicalDomain=Mechanical  PortType=blob  Muxed=off  Pose=off  Angle=on  AngleUnits=rad  ArcVelocity=on  ArcVelocityUnits=rad/s  ArcAcceleration=off  ArcAccelerationUnits=deg/s^2  CoordPosition=on  CoordPositionUnits=m  Velocity=on  VelocityUnits=m/s  Acceleration=off  AccelerationUnits=m/s^2  Quaternion=on  QuaternionDT=off  QuaternionDDT=off  QuaternionUnits=off  OutputVector=[ 1 1 ]  ActiveIO=on  Width=2  DialogClass=MechanicalSensorBlock  Primitive=R1  Force=off  ForceUnits=N  Torque=off  TorqueUnits=N-m  ReferenceFrame=Absolute (INERTIAL)  ReactionSensedSide=Base  ReactionReferenceFrame=Absolute (World)  ReactionForce=off  ReactionForceUnits=N  ReactionMoment=off  ReactionMomentUnits=N-m
  Right Hip IC : mblibv1/Sensors &  Actuators/Joint Initial Condition  UpdateFromCAD=off  LeftPortType=blob  RightPortType=blob  PhysicalDomain=mechanical  DialogClass=InitialConditionBlock  InitialConditions=P1$false$0$m$rad$0$m/s$rad/s#P2$false$0$m$rad$0$m/s$rad/s#P3$false$0$m$rad$0$m/s$rad/s#R1$true$Rphi340$m$rad$0$m/s$rad/s#R2$false$0$m$rad$0$m/s$rad/s#R3$false$0$m$rad$0$m/s$rad/s#S$false$0$m$rad$0$m/s$rad/s  P1PIC=0  P1VIC=0  P2PIC=0  P2VIC=0  P3PIC=0  P3VIC=0  R1PIC=Rphi340  R1VIC=0  R2PIC=0  R2VIC=0  R3PIC=0  R3VIC=0  SPIC=0  SVIC=0
  Right Knee Actuator : mblibv1/Sensors &  Actuators/Joint Actuator  UpdateFromCAD=off  PhysicalDomain=Mechanical  PortType=blob  ActuationStyle=Force  AngleUnits=deg  ArcVelocityUnits=deg/s  ArcAccelerationUnits=deg/s^2  CoordPositionUnits=m  VelocityUnits=m/s  AccelerationUnits=m/s^2  ForceUnits=N  TorqueUnits=N-m  ActiveIO=on  Width=1  DialogClass=MechanicalActuatorBlock  Primitive=R1  ReferenceFrame=Absolute (INERTIAL)
  Right Knee Sensor : mblibv1/Sensors &  Actuators/Joint Sensor  UpdateFromCAD=off  PhysicalDomain=Mechanical  PortType=blob  Muxed=off  Pose=off  Angle=on  AngleUnits=rad  ArcVelocity=on  ArcVelocityUnits=rad/s  ArcAcceleration=off  ArcAccelerationUnits=deg/s^2  CoordPosition=on  CoordPositionUnits=m  Velocity=off  VelocityUnits=m/s  Acceleration=off  AccelerationUnits=m/s^2  Quaternion=on  QuaternionDT=off  QuaternionDDT=off  QuaternionUnits=off  OutputVector=[ 1 1 ]  ActiveIO=on  Width=2  DialogClass=MechanicalSensorBlock  Primitive=R1  Force=off  ForceUnits=N  Torque=off  TorqueUnits=N-m  ReferenceFrame=Absolute (INERTIAL)  ReactionSensedSide=Base  ReactionReferenceFrame=Absolute (World)  ReactionForce=off  ReactionForceUnits=N  ReactionMoment=off  ReactionMomentUnits=N-m
  Right Knee IC : mblibv1/Sensors &  Actuators/Joint Initial Condition  UpdateFromCAD=off  LeftPortType=blob  RightPortType=blob  PhysicalDomain=mechanical  DialogClass=InitialConditionBlock  InitialConditions=P1$false$0$m$rad$0$m/s$rad/s#P2$false$0$m$rad$0$m/s$rad/s#P3$false$0$m$rad$0$m/s$rad/s#R1$true$Rphi230$m$rad$0$m/s$rad/s#R2$false$0$m$rad$0$m/s$rad/s#R3$false$0$m$rad$0$m/s$rad/s#S$false$0$m$rad$0$m/s$rad/s  P1PIC=0  P1VIC=0  P2PIC=0  P2VIC=0  P3PIC=0  P3VIC=0  R1PIC=Rphi230  R1VIC=0  R2PIC=0  R2VIC=0  R3PIC=0  R3VIC=0  SPIC=0  SVIC=0
  Right Leg Load : Subsystem
  Right Shank : mblibv1/Bodies/Body  LConnTagsString=CS3|CS1  RConnTagsString=CS2  UpdateFromCAD=off  DialogClass=MechanicalBodyBlock  Mass=m_S  MassUnits=kg  InertiaUnits=kg*m^2  Inertia=[0 0 0; 0 0 0; 0 0 In_S]  Shape=Cylinder  ShapeDims=[1 1]  ShapeUnits=m  ShapeUse=false  Density=1  DensityUnits=kg/m^3  DensityUse=false  GraphicsMode=MACHINE_DEFAULT  BodyColorSelMode=MACHINE_DEFAULT  BodyColor=[1 0 0]  AttachedToCS=CG  CG=Left$CG$[D1G_S 0 0]$CS1$CS1$m$[0 0 0]$Euler X-Y-Z$deg$WORLD$false$none  WorkingFrames=Left$CS3$[0 0 0]$CS1$CS1$m$[0 0 0]$Euler X-Y-Z$deg$WORLD$true$none#Left$CS1$[0 0 0]$ADJOINING$ADJOINING$m$[0 0 0]$Euler X-Y-Z$deg$WORLD$true$none#Right$CS2$[D12_S 0 0]$CS1$CS1$m$[0 0 0]$Euler X-Y-Z$deg$WORLD$true$none  CGPos=[D1G_S 0 0]  CGRot=[0 0 0]  CS0Pos=[]  CS0Rot=[]  CS1Pos=[0 0 0]  CS1Rot=[0 0 0]  CS2Pos=[D12_S 0 0]  CS2Rot=[0 0 0]  CS3Pos=[0 0 0]  CS3Rot=[0 0 0]  CS4Pos=[]  CS4Rot=[]  CS5Pos=[]  CS5Rot=[]  CS6Pos=[]  CS6Rot=[]  CS7Pos=[]  CS7Rot=[]  CS8Pos=[]  CS8Rot=[]  CS9Pos=[]  CS9Rot=[]  CS10Pos=[]  CS10Rot=[]  CS11Pos=[]  CS11Rot=[]  CS12Pos=[]  CS12Rot=[]  CS13Pos=[]  CS13Rot=[]  CS14Pos=[]  CS14Rot=[]  CS15Pos=[]  CS15Rot=[]  CS16Pos=[]  CS16Rot=[]  CS17Pos=[]  CS17Rot=[]  CS18Pos=[]  CS18Rot=[]  CS19Pos=[]  CS19Rot=[]  CS20Pos=[]  CS20Rot=[]
  Right Thigh Sensor Sheet : Subsystem
  Right Thigh High : mblibv1/Bodies/Body  LConnTagsString=CS2  RConnTagsString=CS1  UpdateFromCAD=off  DialogClass=MechanicalBodyBlock  Mass=m_T*(1-ThPos)  MassUnits=kg  InertiaUnits=kg*m^2  Inertia=[0 0 0; 0 0 0; 0 0 In_T*(1-ThPos)^3]  Shape=Cylinder  ShapeDims=[1 1]  ShapeUnits=m  ShapeUse=false  Density=1  DensityUnits=kg/m^3  DensityUse=false  GraphicsMode=MACHINE_DEFAULT  BodyColorSelMode=MACHINE_DEFAULT  BodyColor=[1;0;0]  AttachedToCS=CG  CG=Left$CG$[-D1G_T*(1-ThPos) 0 0]$CS1$CS1$m$[0 0 0]$Euler X-Y-Z$deg$WORLD$false  WorkingFrames=Right$CS1$[0 0 0]$ADJOINING$ADJOINING$m$[0 0 0]$Euler X-Y-Z$deg$WORLD$true#Left$CS2$[-D12_T*(1-ThPos) 0 0]$CS1$CS1$m$[0 0 0]$Euler X-Y-Z$deg$WORLD$true  CGPos=[-D1G_T*(1-ThPos) 0 0]  CGRot=[0 0 0]  CS0Pos=[]  CS0Rot=[]  CS1Pos=[0 0 0]  CS1Rot=[0 0 0]  CS2Pos=[-D12_T*(1-ThPos) 0 0]  CS2Rot=[0 0 0]  CS3Pos=[]  CS3Rot=[]  CS4Pos=[]  CS4Rot=[]  CS5Pos=[]  CS5Rot=[]  CS6Pos=[]  CS6Rot=[]  CS7Pos=[]  CS7Rot=[]  CS8Pos=[]  CS8Rot=[]  CS9Pos=[]  CS9Rot=[]  CS10Pos=[]  CS10Rot=[]  CS11Pos=[]  CS11Rot=[]  CS12Pos=[]  CS12Rot=[]  CS13Pos=[]  CS13Rot=[]  CS14Pos=[]  CS14Rot=[]  CS15Pos=[]  CS15Rot=[]  CS16Pos=[]  CS16Rot=[]  CS17Pos=[]  CS17Rot=[]  CS18Pos=[]  CS18Rot=[]  CS19Pos=[]  CS19Rot=[]  CS20Pos=[]  CS20Rot=[]
  Right Thigh Low : mblibv1/Bodies/Body  LConnTagsString=CS2  RConnTagsString=CS3|CS1  UpdateFromCAD=off  DialogClass=MechanicalBodyBlock  Mass=m_T*ThPos  MassUnits=kg  InertiaUnits=kg*m^2  Inertia=[0 0 0; 0 0 0; 0 0 In_T*(ThPos)^3]  Shape=Cylinder  ShapeDims=[1 1]  ShapeUnits=m  ShapeUse=false  Density=1  DensityUnits=kg/m^3  DensityUse=false  GraphicsMode=MACHINE_DEFAULT  BodyColorSelMode=MACHINE_DEFAULT  BodyColor=[1 0 0]  AttachedToCS=CG  CG=Left$CG$[-D1G_T*ThPos 0 0]$CS1$CS1$m$[0 0 0]$Euler X-Y-Z$deg$WORLD$false$none  WorkingFrames=Right$CS3$[0 0 0]$CS1$CS1$m$[0 0 0]$Euler X-Y-Z$deg$WORLD$true$none#Right$CS1$[0 0 0]$ADJOINING$ADJOINING$m$[0 0 0]$Euler X-Y-Z$deg$WORLD$true$none#Left$CS2$[-D12_T*ThPos 0 0]$CS1$CS1$m$[0 0 0]$Euler X-Y-Z$deg$WORLD$true$none  CGPos=[-D1G_T*ThPos 0 0]  CGRot=[0 0 0]  CS0Pos=[]  CS0Rot=[]  CS1Pos=[0 0 0]  CS1Rot=[0 0 0]  CS2Pos=[-D12_T*ThPos 0 0]  CS2Rot=[0 0 0]  CS3Pos=[0 0 0]  CS3Rot=[0 0 0]  CS4Pos=[]  CS4Rot=[]  CS5Pos=[]  CS5Rot=[]  CS6Pos=[]  CS6Rot=[]  CS7Pos=[]  CS7Rot=[]  CS8Pos=[]  CS8Rot=[]  CS9Pos=[]  CS9Rot=[]  CS10Pos=[]  CS10Rot=[]  CS11Pos=[]  CS11Rot=[]  CS12Pos=[]  CS12Rot=[]  CS13Pos=[]  CS13Rot=[]  CS14Pos=[]  CS14Rot=[]  CS15Pos=[]  CS15Rot=[]  CS16Pos=[]  CS16Rot=[]  CS17Pos=[]  CS17Rot=[]  CS18Pos=[]  CS18Rot=[]  CS19Pos=[]  CS19Rot=[]  CS20Pos=[]  CS20Rot=[]
  Terminator1 : Terminator
  Terminator4 : Terminator
  map (-pi,pi] to [0,2pi){,3..7} (6 alike) : Fcn  Expr=u*(u>=0) + (2*pi+u)*(u<0)
  tag scope: LBallCnt=global, LHeelCnt=global, LKneeState=global, LLLoad=global, LdxThigh=global, Lphi12dphi12=global, Lphi23dphi23=global, Lphi34dphi34=global, RBallCnt=global, RHeelCnt=global, RKneeState=global, RLLoad=global, RdxThigh=global, Rphi12dphi12=global, Rphi23dphi23=global, Rphi34dphi34=global, dxyzHAT=global, dxyzLHip=global, dxyzRHip=global, rotTrunk=global, xyzHAT=global, xyzLAnkle=global, xyzLBall=global, xyzLHeel=global, xyzLHip=global, xyzLKnee=global, xyzRAnkle=global, xyzRBall=global, xyzRHeel=global, xyzRHip=global, xyzRKnee=global, xyzTrunk=global
  wires:
  [RStance] -> Right Force Plate/Enable
  Right Heel Contact1/2(GRF [N N]) -> Right Force Plate/1("GRF_Ball [N N] ")
  Right Heel Contact/2(GRF [N N]) -> Right Force Plate/2(GRF_Heel [N N])
  Right Force Plate/1(GRFs) -> Demux/1
  Demux/1 -> R_GRF/1
  Demux/2 -> R_GRF/2
  Demux/3 -> R_GRF/3
  Right Force Plate/2(COP) -> Terminator4/1
  Right Heel Sensor5/1 -> [xyzHAT]
  Right Heel Sensor5/2 -> [dxyzHAT]
  [LStance] -> Left Force Plate/Enable
  Right Heel Contact3/2(GRF [N N]) -> Left Force Plate/1("GRF_Ball [N N] ")
  Right Heel Contact2/2(GRF [N N]) -> Left Force Plate/2(GRF_Heel [N N])
  Left Force Plate/1(GRFs) -> Demux1/1
  Demux1/1 -> L_GRF/1
  Demux1/2 -> L_GRF/2
  Demux1/3 -> L_GRF/3
  Left Force Plate/2(COP) -> Terminator1/1
  [RM12] -> Right Ankle Actuator/1
  [RM23] -> Right Knee Actuator/1
  [RM34] -> Right Hip Actuator/1
  [LM12] -> Left Ankle Actuator/1
  [LM23] -> Left Knee Actuator/1
  [LM34] -> Left Hip Actuator/1
  Right Heel Sensor9/1 -> [xyzLHip]
  Right Heel Sensor9/2 -> [dxyzLHip]
  Right Heel Sensor8/2 -> [dxyzRHip]
  Right Heel Sensor8/1 -> [xyzRHip]
  Right Heel Contact2/1(RHeelCnt) -> L Heel Skin Load Sensor/1
  L Heel Skin Load Sensor/1 -> [LHeelCnt]
  L Ball Skin Load Sensor/1 -> [LBallCnt]
  Right Heel Contact3/1(RHeelCnt) -> L Ball Skin Load Sensor/1
  R Heel Skin Load Sensor/1 -> [RHeelCnt]
  Right Heel Contact/1(RHeelCnt) -> R Heel Skin Load Sensor/1
  Right Heel Contact1/1(RHeelCnt) -> R Ball Skin Load Sensor/1
  R Ball Skin Load Sensor/1 -> [RBallCnt]
  Left Thigh Sensor Sheet/1(dx) -> L Thigh Displacement  Sensor/1
  L Thigh Displacement  Sensor/1 -> Left Leg Load/1(dxThigh [m]), [LdxThigh]
  Right Thigh Sensor Sheet/1(dx) -> R Thigh Displacement  Sensor/1
  R Thigh Displacement  Sensor/1 -> Right Leg Load/1(dxThigh [m]), [RdxThigh]
  map (-pi,pi] to [0,2pi)/1 -> Mux2/1
  Left Hip Sensor/2 -> Mux2/2
  Left Hip Sensor/1 -> map (-pi,pi] to [0,2pi)/1
  Mux2/1 -> [Lphi34dphi34]
  map (-pi,pi] to [0,2pi)5/1 -> Mux3/1
  Right Hip Sensor/2 -> Mux3/2
  Right Hip Sensor/1 -> map (-pi,pi] to [0,2pi)5/1
  Mux3/1 -> [Rphi34dphi34]
  map (-pi,pi] to [0,2pi)6/1 -> Mux4/1
  LeftKnee Sensor/2 -> Mux4/2
  LeftKnee Sensor/1 -> map (-pi,pi] to [0,2pi)6/1
  Mux4/1 -> [Lphi23dphi23], L Knee Joint Sensor/1
  map (-pi,pi] to [0,2pi)4/1 -> Mux5/1
  Right Knee Sensor/2 -> Mux5/2
  Mux5/1 -> [Rphi23dphi23], R Knee Joint Sensor/1
  Right Knee Sensor/1 -> map (-pi,pi] to [0,2pi)4/1
  map (-pi,pi] to [0,2pi)3/1 -> Mux6/1
  Left Ankle Sensor/2 -> Mux6/2
  Left Ankle Sensor/1 -> map (-pi,pi] to [0,2pi)3/1
  Mux6/1 -> [Lphi12dphi12]
  map (-pi,pi] to [0,2pi)7/1 -> Mux7/1
  Right Ankle Sensor/2 -> Mux7/2
  Right Ankle Sensor/1 -> map (-pi,pi] to [0,2pi)7/1
  Mux7/1 -> [Rphi12dphi12]
  L Knee Joint Sensor/1 -> [LKneeState]
  R Knee Joint Sensor/1 -> [RKneeState]
  Right Heel Sensor1/1 -> [xyzRKnee]
  Right Heel Sensor2/1 -> [xyzLKnee]
  Right Heel Sensor3/1 -> [xyzLAnkle]
  Right Heel Sensor4/1 -> [xyzRAnkle]
  Left Leg Load/1(LLoad [F]) -> [LLLoad]
  Right Leg Load/1(LLoad [F]) -> [RLLoad]
  Right Heel Sensor7/1 -> [xyzLHeel]
  Right Heel Sensor10/1 -> [xyzLBall]
  Right Heel Sensor12/1 -> [xyzRHeel]
  Right Heel Sensor11/1 -> [xyzRBall]
  [xyzHAT_D_sag] -> RLBall Cnt1/1(Dist_sag)
  RLBall Cnt1/1(Pos) -> [xyzTrunk]
  RLBall Cnt1/2(Rot) -> [rotTrunk]
  connections:
  HAT/RConn1 -- Left Hip Joint/RConn1
  Left Foot/RConn1 -- Left Ankle Joint/LConn1
  Left Ankle Joint/LConn2 -- Left Ankle Actuator/RConn1
  Left Ankle Sensor/LConn1 -- Left Ankle Joint/LConn3
  Left Ankle Joint/RConn1 -- Left Shank/LConn2
  Left Ankle Joint/RConn2 -- Left Ankle IC/RConn1
  Right Heel Contact2/LConn1 -- Left Foot/RConn2
  Left Hip Joint/LConn1 -- Left Thigh High/LConn1
  Left Hip Joint/LConn2 -- Left Hip Actuator/RConn1
  Left Hip Joint/LConn3 -- Left Hip Sensor/LConn1
  Left Hip Joint/RConn2 -- Left Hip IC/RConn1
  Left Shank/RConn1 -- Left Knee Joint/LConn1
  Left Knee Joint/LConn2 -- Left Knee Actuator/RConn1
  LeftKnee Sensor/LConn1 -- Left Knee Joint/LConn3
  Left Knee Joint/RConn1 -- Left Thigh Low/RConn2
  Left Knee Joint/RConn2 -- Left Knee IC/RConn1
  Left Thigh Sensor Sheet/LConn1 -- Left Thigh Low/LConn1
  Left Thigh High/RConn1 -- Left Thigh Sensor Sheet/RConn1
  Right Foot/RConn1 -- Right Ankle Joint/LConn1
  Right Ankle Actuator/RConn1 -- Right Ankle Joint/LConn2
  Right Ankle Joint/LConn3 -- Right Ankle Sensor/LConn1
  Right Ankle Joint/RConn1 -- Right Shank/LConn2
  Right Ankle Joint/RConn2 -- Right Ankle IC/RConn1
  Right Heel Contact1/LConn1 -- Right Foot/LConn1
  Right Heel Contact/LConn1 -- Right Foot/RConn2
  Right Hip Joint/LConn1 -- Right Thigh High/LConn1
  Right Hip Joint/LConn2 -- Right Hip Actuator/RConn1
  Right Hip Joint/LConn3 -- Right Hip Sensor/LConn1
  Right Hip IC/RConn1 -- Right Hip Joint/RConn2
  Right Shank/RConn1 -- Right Knee Joint/LConn1
  Right Knee Actuator/RConn1 -- Right Knee Joint/LConn2
  Right Knee Joint/LConn3 -- Right Knee Sensor/LConn1
  Right Knee Joint/RConn1 -- Right Thigh Low/RConn2
  Right Knee Joint/RConn2 -- Right Knee IC/RConn1
  Right Thigh Sensor Sheet/LConn1 -- Right Thigh Low/LConn1
  Right Thigh High/RConn1 -- Right Thigh Sensor Sheet/RConn1
  HAT/RConn2 -- Right Heel Sensor9/LConn1
  Right Heel Sensor5/LConn1 -- HAT/LConn1
  Ground/LConn1 -- Machine Environment/RConn1
  Right Heel Contact3/LConn1 -- Left Foot/LConn2
  Planar/LConn1 -- Ground/RConn1
  Planar/RConn1 -- Left Foot/LConn1
  HAT/RConn4 -- Right Hip Joint/RConn1
  HAT/RConn3 -- Right Heel Sensor8/LConn1
  Planar/LConn2 -- Left Ball IC/RConn1
  Right Heel Sensor1/LConn1 -- Right Thigh Low/RConn1
  Right Heel Sensor2/LConn1 -- Left Thigh Low/RConn1
  Right Heel Sensor3/LConn1 -- Left Shank/LConn1
  Right Heel Sensor4/LConn1 -- Right Shank/LConn1
  HAT/LConn2 -- RLBall Cnt1/LConn1
  Right Heel Sensor7/LConn1 -- Left Foot/RConn3
  Left Foot/LConn3 -- Right Heel Sensor10/LConn1
  Right Heel Sensor12/LConn1 -- Right Foot/RConn3
  Right Heel Sensor11/LConn1 -- Right Foot/LConn2

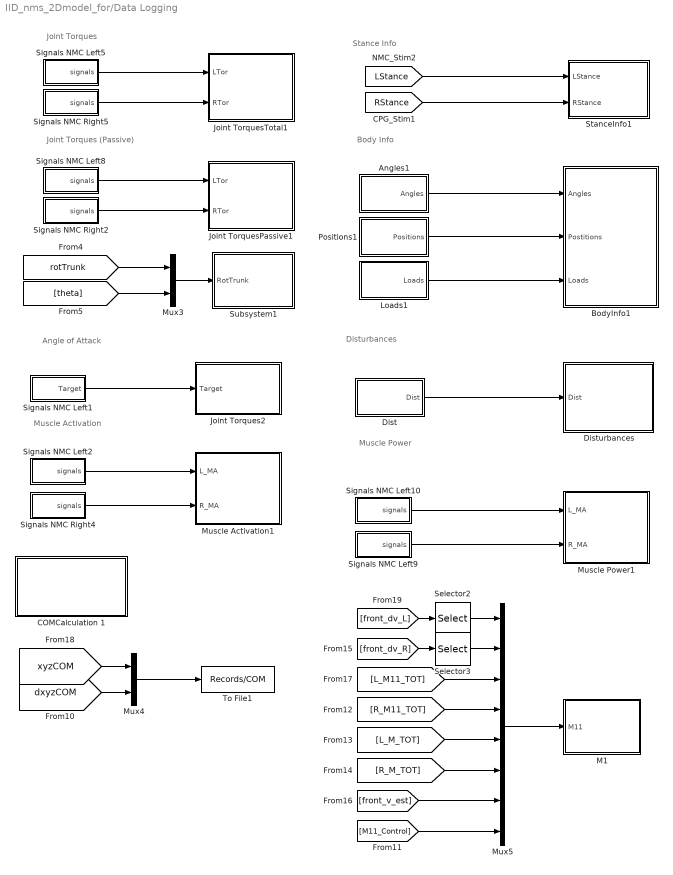
== system IID_nms_2Dmodel_for/Data Logging ==
  note: Disturbances
  note: Stance Info
  note: Muscle Activation
  note: Joint Torques
  note: Angle of Attack
  note: Body Info
  note: Joint Torques (Passive)
  note: Muscle Power
  Angles1 : Subsystem
  BodyInfo1 : Subsystem
  COMCalculation 1 : Subsystem
  Dist : Subsystem
  Disturbances : Subsystem
  Joint Torques2 : Subsystem
  Joint TorquesPassive1 : Subsystem
  Joint TorquesTotal1 : Subsystem
  Loads1 : Subsystem
  M1 : Subsystem
  Muscle Activation1 : Subsystem
  Muscle Power1 : Subsystem
  Mux3 : Mux  Inputs=2
  Mux4 : Mux  Inputs=2
  Mux5 : Mux  Inputs=8
  Positions1 : Subsystem
  Selector2 : Selector  InputPortWidth=2  IndexOptions=Index vector (dialog)  Indices=[2]  OutputSizes=1
  Selector3 : Selector  InputPortWidth=2  IndexOptions=Index vector (dialog)  Indices=[2]  OutputSizes=1
  Signals NMC Left1 : Subsystem
  Signals NMC Left10 : Subsystem
  Signals NMC Left2 : Subsystem
  Signals NMC Left5 : Subsystem
  Signals NMC Left8 : Subsystem
  Signals NMC Left9 : Subsystem
  Signals NMC Right2 : Subsystem
  Signals NMC Right4 : Subsystem
  Signals NMC Right5 : Subsystem
  StanceInfo1 : Subsystem
  Subsystem1 : Subsystem
  To File1 : ToFile  Filename=Records/COM
  wires:
  Dist/1(Dist) -> Disturbances/1(Dist)
  Signals NMC Right4/1(signals) -> Muscle Activation1/2(R_MA)
  Signals NMC Left2/1(signals) -> Muscle Activation1/1(L_MA)
  Signals NMC Left5/1(signals) -> Joint TorquesTotal1/1(LTor)
  Signals NMC Right5/1(signals) -> Joint TorquesTotal1/2(RTor)
  Angles1/1(Angles) -> BodyInfo1/1(Angles)
  Positions1/1(Positions) -> BodyInfo1/2(Postitions)
  [LStance] -> StanceInfo1/1(LStance)
  [RStance] -> StanceInfo1/2(RStance)
  Loads1/1(Loads) -> BodyInfo1/3(Loads)
  Signals NMC Left1/1(Target) -> Joint Torques2/1(Target)
  [rotTrunk] -> Mux3/1
  [theta] -> Mux3/2
  Signals NMC Left8/1(signals) -> Joint TorquesPassive1/1(LTor)
  Signals NMC Right2/1(signals) -> Joint TorquesPassive1/2(RTor)
  Signals NMC Left9/1(signals) -> Muscle Power1/2(R_MA)
  Signals NMC Left10/1(signals) -> Muscle Power1/1(L_MA)
  Mux3/1 -> Subsystem1/1(RotTrunk)
  [dxyzCOM] -> Mux4/2
  [xyzCOM] -> Mux4/1
  Mux4/1 -> To File1/1
  Selector2/1 -> Mux5/1
  [front_dv_L] -> Selector2/1
  [L_M_TOT] -> Mux5/5
  [R_M_TOT] -> Mux5/6
  [L_M11_TOT] -> Mux5/3
  [R_M11_TOT] -> Mux5/4
  [front_dv_R] -> Selector3/1
  Selector3/1 -> Mux5/2
  Mux5/1 -> M1/1(M11)
  [M11_Control] -> Mux5/8
  [front_v_est] -> Mux5/7

== system IID_nms_2Dmodel_for/Disturbances ==
  Clock : Clock
  Compare To Constant : simulink/Logic and Bit Operations/Compare To Constant  relop=>  const=Dist_StartTime  OutDataTypeStr=boolean
  Compare To Constant1 : simulink/Logic and Bit Operations/Compare To Constant  relop===  const=0  OutDataTypeStr=boolean
  Compare To Constant2 : simulink/Logic and Bit Operations/Compare To Constant  relop===  const=1  OutDataTypeStr=boolean
  Compare To Constant3 : simulink/Logic and Bit Operations/Compare To Constant  relop=<  const=Dist_PDur  OutDataTypeStr=boolean
  Constant : Constant  Value=0
  Constant1 : Constant  Value=Dist_On
  Constant2 : Constant  Value=Dist_xyzHAT_sag_PH
  Disturbances : Subsystem
  Integrator : Integrator
  Logical Operator : Logic  Inputs=4  AllPortsSameDT=off  OutDataTypeStr=boolean
  Logical Operator1 : Logic  AllPortsSameDT=off  OutDataTypeStr=boolean
  SampleAndHold : Subsystem
  Start Disturbance torques onces CPG is turned on : Switch  Criteria=u2 ~= 0
  Transport Delay1 : TransportDelay  DelayTime=0.01
  wires:
  Constant1/1 -> Logical Operator/2
  Compare To Constant/1 -> Logical Operator/1
  Constant2/1 -> Start Disturbance torques onces CPG is turned on/1
  Start Disturbance torques onces CPG is turned on/1 -> Disturbances/1(Dist)
  Constant/1 -> Start Disturbance torques onces CPG is turned on/3
  Clock/1 -> Compare To Constant/1
  Compare To Constant1/1 -> Logical Operator/3
  [LStance] -> Compare To Constant1/1, Transport Delay1/1
  Compare To Constant2/1 -> Logical Operator/4
  Logical Operator1/1 -> Start Disturbance torques onces CPG is turned on/2
  Transport Delay1/1 -> Compare To Constant2/1
  Integrator/1 -> Compare To Constant3/1
  Compare To Constant3/1 -> Logical Operator1/2
  SampleAndHold/1(Out) -> Logical Operator1/1, Integrator/1
  Logical Operator/1 -> SampleAndHold/1(Sample), SampleAndHold/2(Value)

== system IID_nms_2Dmodel_for/Full Body Control ==
  note: NMC MAIN CONTROL
  EnableJointLimits : Constant  OutDataTypeStr=double
      settings: OpenFcn=|
      | b = get_param(gcb,'value');
      | if (strcmp(b,'1')),
      |   set_param (gcb,'value','0');
      | else
      |   set_param(gcb,'value','1');
      | end;
  Left Side : Subsystem
  Main Control Goto : Subsystem
  Right Side : Subsystem
  Sensors : Subsystem
  tag scope: LM12=global, LM23=global, LM34=global, RM12=global, RM23=global, RM34=global
  wires:
  [Lphi34dphi34] -> Left Side/1(LphidphiHip)
  [Lphi23dphi23] -> Left Side/2(LphidphiKnee)
  Left Side/1(LTauHip) -> [LM34]
  Left Side/2(LTauKnee) -> [LM23]
  Left Side/3(LTauAnkle) -> [LM12]
  [Lphi12dphi12] -> Left Side/3(LphidphiAnkle)
  [Rphi34dphi34] -> Right Side/1(RphidphiHip)
  [Rphi23dphi23] -> Right Side/2(RphidphiKnee)
  [Rphi12dphi12] -> Right Side/3(RphidphiAnkle)
  Right Side/1(RTauHip) -> [RM34]
  Right Side/2(RTauKnee) -> [RM23]
  Right Side/3(RTauAnkle) -> [RM12]
  EnableJointLimits/1 -> Main Control Goto/1(EnableNMC_JointLimits)

== system IID_nms_2Dmodel_for/Positions ==
  Mux : Mux  Inputs=11
  Positions : Outport
  wires:
  Mux/1 -> Positions/1
  [xyzRAnkle] -> Mux/7
  [xyzLKnee] -> Mux/4
  [xyzLHip] -> Mux/5
  [dxyzLHip] -> Mux/6
  [xyzRKnee] -> Mux/8
  [xyzLAnkle] -> Mux/3
  [xyzRHip] -> Mux/9
  [dxyzRHip] -> Mux/10
  [xyzHAT] -> Mux/1
  [dxyzHAT] -> Mux/2
  [xyzTrunk] -> Mux/11

== system IID_nms_2Dmodel_for/Signals NMC Left3 ==
  Mux : Mux
  signals : Outport
  wires:
  Mux/1 -> signals/1
  [LM34] -> Mux/1
  [LM23] -> Mux/3
  [LM12] -> Mux/4
  [LM34R] -> Mux/2

== system IID_nms_2Dmodel_for/Signals NMC Left6 ==
  Mux : Mux  Inputs=7
  signals : Outport
  wires:
  Mux/1 -> signals/1
  [REnergyVAS] -> Mux/2
  [REnergyHFL] -> Mux/1
  [REnergyTA] -> Mux/3
  [REnergySOL] -> Mux/4
  [REnergyHAM] -> Mux/6
  [REnergyGAS] -> Mux/5
  [REnergyGLU] -> Mux/7
